simulink library "AngleOfRotation"  (R2018a)
settings: Solver=VariableStepAuto  StartTime=0.0  StopTime=10.0  RelTol=1e-3
libraries: simulink_extras x2
settings Model: Creator=rahul  LastModifiedBy=rahul

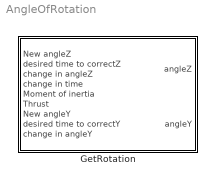
== system AngleOfRotation ==
  GetRotation : Subsystem

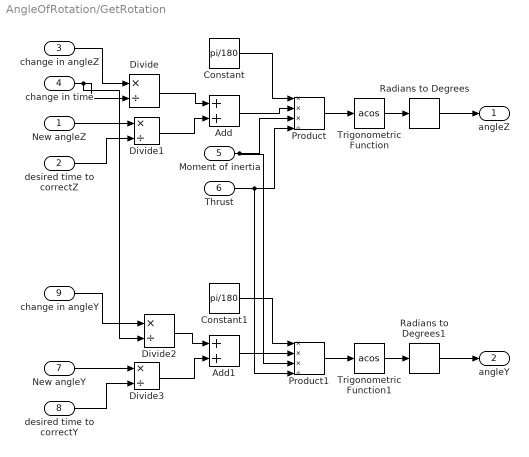
== system AngleOfRotation/GetRotation ==
  New angleZ : Inport
  desired time to correctZ : Inport  Port=2
  change in angleZ : Inport  Port=3
  change in time : Inport  Port=4
  Moment of inertia : Inport  Port=5
  Thrust : Inport  Port=6
  New angleY : Inport  Port=7
  desired time to correctY : Inport  Port=8
  change in angleY : Inport  Port=9
  Add : Sum
  Add1 : Sum
  Constant : Constant  Value=pi/180
  Constant1 : Constant  Value=pi/180
  Divide{,1..3} (4 alike) : Product  Inputs=*/
  Product : Product  Inputs=***/
  Product1 : Product  Inputs=***/
  Radians to Degrees : simulink_extras/Transformations/Radians to Degrees
  Radians to Degrees1 : simulink_extras/Transformations/Radians to Degrees
  Trigonometric Function : Trigonometry  Operator=acos
  Trigonometric Function1 : Trigonometry  Operator=acos
  angleZ : Outport
  angleY : Outport  Port=2
  wires:
  change in angleZ/1 -> Divide/1
  Add/1 -> Product/2
  Product/1 -> Trigonometric Function/1
  Divide1/1 -> Add/2
  Constant/1 -> Product/1
  desired time to correctZ/1 -> Divide1/2
  Radians to Degrees/1 -> angleZ/1
  Divide/1 -> Add/1
  New angleZ/1 -> Divide1/1
  Trigonometric Function/1 -> Radians to Degrees/1
  desired time to correctY/1 -> Divide3/2
  change in time/1 -> Divide2/2, Divide/2
  Divide3/1 -> Add1/2
  Trigonometric Function1/1 -> Radians to Degrees1/1
  Thrust/1 -> Product1/4, Product/4
  New angleY/1 -> Divide3/1
  Constant1/1 -> Product1/1
  Product1/1 -> Trigonometric Function1/1
  Divide2/1 -> Add1/1
  Radians to Degrees1/1 -> angleY/1
  change in angleY/1 -> Divide2/1
  Moment of inertia/1 -> Product1/3, Product/3
  Add1/1 -> Product1/2
